simulink model "without-attack"  (R2018b)
settings: Solver=VariableStepAuto  StartTime=0.0  StopTime=5  RelTol=1e-3
undefined symbols (not defined in the file or in its folder): Ts
settings Model: Creator=lenovo  LastModifiedBy=lenovo

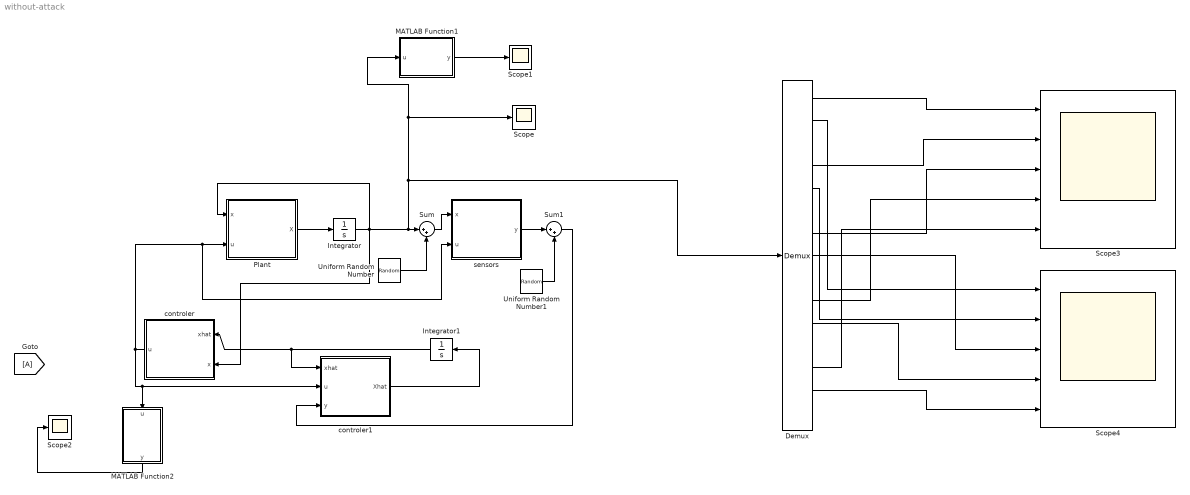
== system without-attack ==
  Demux : Demux  Outputs=15
  Integrator : Integrator  InitialCondition=[-7;-6;-5;-4;-3;-2;-1;0;1;2;3;4;5;6;7]
  Integrator1 : Integrator  InitialCondition=[-7;-6;-5;-4;-3;-2;-1;0;1;2;3;4;5;6;7]
  MATLAB Function1 : MATLAB Function  TreatAsAtomicUnit=on
  MATLAB Function2 : MATLAB Function  TreatAsAtomicUnit=on
  Plant : MATLAB Function  TreatAsAtomicUnit=on
  Scope : Scope
  Scope1 : Scope
  Scope2 : Scope
  Scope3 : Scope  NumInputPorts=5
  Scope4 : Scope  NumInputPorts=5
  Sum : Sum  Inputs=|++
  Sum1 : Sum  Inputs=|++
  Uniform Random Number : UniformRandomNumber  Minimum=-0.01  Maximum=0.01  SampleTime=Ts
  Uniform Random Number1 : UniformRandomNumber  Minimum=-0.01  Maximum=0.01  SampleTime=Ts
  controler : MATLAB Function  TreatAsAtomicUnit=on
  controler1 : MATLAB Function  TreatAsAtomicUnit=on
  sensors : MATLAB Function  TreatAsAtomicUnit=on
  wires:
  Integrator1/1 -> controler1/1(xhat), controler/1(xhat)
  sensors/1(y) -> Sum1/1
  Sum1/1 -> controler1/3(y)
  Uniform Random Number/1 -> Sum/2
  MATLAB Function1/1(y) -> Scope1/1
  Uniform Random Number1/1 -> Sum1/2
  Sum/1 -> sensors/1(x)
  Plant/1(X) -> Integrator/1
  controler1/1(Xhat) -> Integrator1/1
  controler/1(u) -> MATLAB Function2/1(u), controler1/2(u), sensors/2(u), Plant/2(u)
  Integrator/1 -> controler/2(x), MATLAB Function1/1(u), Scope/1, Demux/1, Sum/1, Plant/1(x)
  Demux/1 -> Scope3/1
  Demux/4 -> Scope3/2
  Demux/7 -> Scope3/3
  Demux/10 -> Scope3/4
  Demux/13 -> Scope3/5
  Demux/2 -> Scope4/1
  Demux/5 -> Scope4/2
  Demux/8 -> Scope4/3
  Demux/11 -> Scope4/4
  Demux/14 -> Scope4/5
  MATLAB Function2/1(y) -> Scope2/1

== matlab function without-attack/sensors ==
  data: x input; y output; u input
function y = fcn(x,u)
A=[-25.7442 -14.1298 -8.6868;16 0 0;0 16 0];
B=[8;0;0];
C=[2.3498 -0.2552 3.3462;3.8307 -3.7641 3.9829;4.4177 -5.2315 4.9];
D=[-.5478;-.4304;-.4304];
C0=kron(eye(5),C);
D0=kron(eye(5),D);
y=C0*x+D0*u;

== matlab function without-attack/Plant ==
  data: x input; u input; X output
function X = fcn(x,u)
A=[-25.7442 -14.1298 -8.6868;16 0 0;0 16 0];
B=[8;0;0];
C=[2.3498 -0.2552 3.3462;3.8307 -3.7641 3.9829;4.4177 -5.2315 4.9];
D=[-.5478;-.4304;-.4304];
A0=kron(eye(5),A);
B0=kron(eye(5),B);
X =A0*x+B0*u;

== matlab function without-attack/controler ==
  data: xhat input; u output; x input
function u = fcn(xhat,x)
K=[1.0766 -.3101 0];
c=0.1;
A=[.9226 -.6330 0;1 0 0;0 1 0];
B=[1;0;0];
L=[ 1 0 0 0 -1; -1 1 0 0 0; -1 0 1 0 0; 0 -1 0 1 0; 0 -1 -1 -1 3];
A0=kron(eye(5),A);
B0=kron(eye(5),B);
z=kron(L,eye(3));
Q=z'*eye(15)*z;
q1=[0.8922   -0.6194         0   -0.0189    0.0085         0   -0.0366    0.0167         0 
   -0.0189    0.0085         0    0.8997   -0.6229         0   -0.0210    0.0097         0
   -0.0366    0.0167         0   -0.0210    0.0097         0    0.8361   -0.5943         0
   -0.0260    0.0119         0   -0.0246    0.0112         0   -0.0263    0.0125         0
   -0.0303    0.0138         0   -0.0241    0.0109         0   -0.0471    0.0215         0];
q2=[-0.0260    0.0119         0   -0.0303    0.0138         0
   -0.0246    0.0112         0   -0.0241    0.0109         0
   -0.0263    0.0125         0   -0.0471    0.0215         0
    0.8517   -0.6016         0   -0.0414    0.0188         0
   -0.0414    0.0188         0    0.8781   -0.6129         0];
q=[q1 q2];
% u=-c*kron(L,K)*xhat;
u=-c*q*xhat;

== matlab function without-attack/controler1 ==
  data: xhat input; u input; Xhat output; y input
function Xhat = fcn(xhat,u,y)
A=[-25.7442 -14.1298 -8.6868;16 0 0;0 16 0];
B=[8;0;0];
C=[2.3498 -0.2552 3.3462;3.8307 -3.7641 3.9829;4.4177 -5.2315 4.9];
D=[-.5478;-.4304;-.4304];
G=[0.0450 .0187 .0338;.0005 .0252 .045;-.0631 -.0445 -.0827];
C0=kron(eye(5),C);
D0=kron(eye(5),D);
A0=kron(eye(5),A);
B0=kron(eye(5),B);
G0=kron(eye(5),G);
yhat=C0*xhat+D0*u;
Xhat=A0*xhat+B0*u+G0*(y-yhat);

== matlab function without-attack/MATLAB Function2 ==
  data: u input; y output
function y = fcn( u)
y=norm(u);

== matlab function without-attack/MATLAB Function1 ==
  data: u input; y output
function y = fcn( u)
y=norm(u);
